simulink model "CustArch_v22"  (R2020a)
settings: Solver=FixedStepDiscrete  StartTime=0.0  StopTime=840000  RelTol=1e-3
undefined symbols (not defined in the file): closed_loop_neuroscience, sqrt_uint32
libraries: hdlsllib x107, simulink x104
(part 2 of 3)

== system CustArch_v22/cust_architecture/process_and_retrieve/spike_detection/LocalMaximaAdaptiveThreshold ==
  filter_output : Inport
  InputState : Inport  Port=2
  write porcessing addr = read from storage addr +1 : Inport  Port=3
  LocalMaxima : Subsystem
  RMS_computation : Subsystem
  local_maxima_out : Outport
  wires:
  filter_output/1 -> RMS_computation/1(filter_output), LocalMaxima/2(filter_output)
  InputState/1 -> RMS_computation/3(InputState), LocalMaxima/3(InputState)
  write porcessing addr = read from storage addr +1/1 -> RMS_computation/2(write porcessing addr = read from storage addr +1), LocalMaxima/4(write porcessing addr = read from storage addr +1)
  LocalMaxima/1(Out1) -> local_maxima_out/1
  RMS_computation/1(adaptive_th) -> LocalMaxima/1(adaptive_th)

== system CustArch_v22/cust_architecture/process_and_retrieve/spike_detection/refractory_period ==
  InputState : Inport
  wr_en : Inport  Port=2
  write porcessing addr = read from storage addr +1 : Inport  Port=3
  rd_addr : Inport  Port=4
  Constant : Constant  OutDataTypeStr=uint16  SampleTime=-1
  Constant1 : Constant  Value=0  OutDataTypeStr=uint16  SampleTime=-1
  Delay : Delay  DelayLength=1  InitialCondition=0
  HDL Counter : hdlsllib/Sources/HDL Counter  CountType=Free running  CountInit=0  CountStep=1  CountMax=2^32  CountFromType=Initial value  CountFrom=0  CountResetPort=off  CountLoadPort=off  CountEnbPort=on  CountDirPort=off  CountDataType=Unsigned  CountWordLen=32  CountFracLen=0  CountSampTime=1
  Logical Operator : Logic  IconShape=distinctive  AllPortsSameDT=off  OutDataTypeStr=boolean
  Sum : Sum  Inputs=+-
  Switch : Switch  Criteria=u2 > Threshold
  Terminator2 : Terminator
  Terminator3 : Terminator
  input_state_AC : simulink/Logic and Bit Operations/Compare To Constant  relop===  const=1  OutDataTypeStr=boolean
  refractory_period : simulink/Logic and Bit Operations/Compare To Constant  relop=>=  const=30  OutDataTypeStr=boolean
  spikes : hdlsllib/HDL RAMs/Dual Port RAM  ram_size=9
      settings: SourceProductBaseCode=SL
  timestamp_before : hdlsllib/HDL RAMs/Dual Port RAM  ram_size=9
      settings: SourceProductBaseCode=SL
  refractory_check : Outport
  spike : Outport  Port=2
  wires:
  timestamp_before/1 -> Terminator2/1
  Delay/1 -> spikes/2, timestamp_before/2
  spikes/2 -> spike/1
  write porcessing addr = read from storage addr +1/1 -> input_state_AC/1, Delay/1, timestamp_before/4
  wr_en/1 -> Switch/2, timestamp_before/3
  timestamp_before/2 -> Sum/2
  rd_addr/1 -> spikes/4
  spikes/1 -> Terminator3/1
  Sum/1 -> refractory_period/1
  InputState/1 -> spikes/3, Logical Operator/2  "read from porcessing"
  refractory_period/1 -> Logical Operator/1
  Logical Operator/1 -> refractory_check/1
  input_state_AC/1 -> HDL Counter/1  "read from porcessing"
  HDL Counter/1 -> timestamp_before/1, Sum/1
  Constant/1 -> Switch/1
  Switch/1 -> spikes/1
  Constant1/1 -> Switch/3

== system CustArch_v22/cust_architecture/input_interpret_store_retrieve/Interpret_to_RAM_input/interpret incoming data/condition to count DAC or ADC  ==
  fifo_write_to : Inport
  input_state : Inport  Port=2
  AND : Logic  IconShape=distinctive  AllPortsSameDT=off  OutDataTypeStr=boolean
  OR : Logic  Operator=OR  IconShape=distinctive  AllPortsSameDT=off  OutDataTypeStr=boolean
  is state_ADC : simulink/Logic and Bit Operations/Compare To Constant  relop===  const=13  OutDataTypeStr=boolean
  is state_DAC : simulink/Logic and Bit Operations/Compare To Constant  relop===  const=12  OutDataTypeStr=boolean
  Out1 : Outport  VectorParamsAs1DForOutWhenUnconnected=off
  wires:
  input_state/1 -> is state_DAC/1, is state_ADC/1
  is state_DAC/1 -> OR/1
  is state_ADC/1 -> OR/2
  fifo_write_to/1 -> AND/1
  OR/1 -> AND/2
  AND/1 -> Out1/1

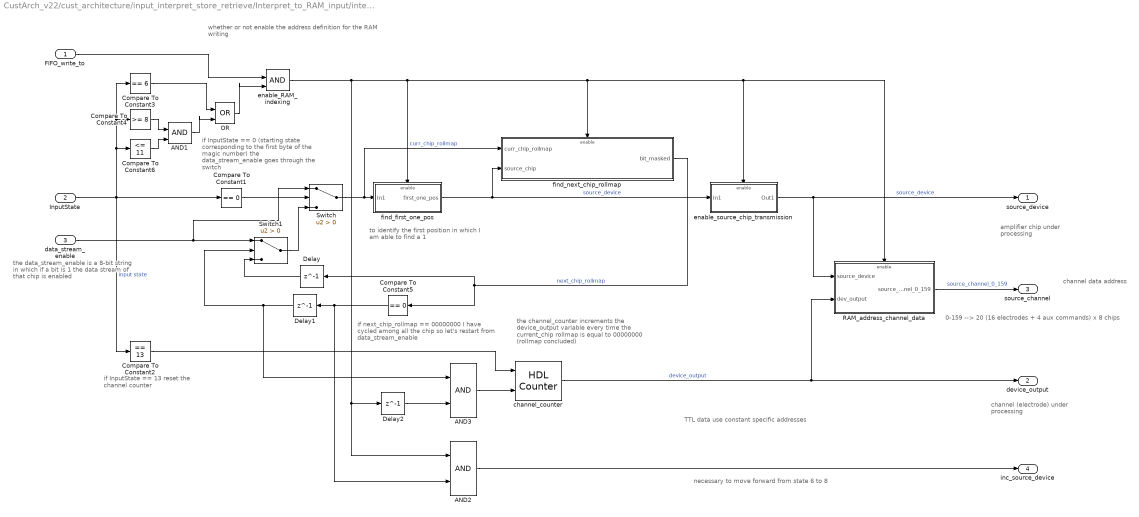
== system CustArch_v22/cust_architecture/input_interpret_store_retrieve/Interpret_to_RAM_input/interpret incoming data/get_sources_and_RAM_addresses ==
  note: necessary to move forward from state 6 to 8
  note: amplifier chip under
      | processing
  note: the channel_counter increments the
      | device_output variable every time the
      | current_chip rollmap is equal to 00000000
      | (rollmap concluded)
  note: if InputState == 13
      | reset the channel counter
  note: whether or not enable the address definition
      | for the RAM writing
  note: if InputState == 0 (starting state corresponding to the first byte
      | of the magic number) the data_stream_enable goes through the switch
  note: 0-159 --> 20 (16 electrodes + 4 aux commands) x 8 chips
  note: to identify the first position in which
      | I am able to find a 1
  note: if next_chip_rollmap == 00000000 I have cycled among all the chip so let's restart from data_stream_enable
  note: the data_stream_enable is a 8-bit string in which if a bit is 1 the data stream of that chip is enabled
  note: channel (electrode) under
      | processing
  note: channel data
      | address
  note: TTL data use constant specific addresses
  FIFO_write_to : Inport
  InputState : Inport  Port=2
  data_stream_enable : Inport  Port=3
  AND1 : Logic  IconShape=distinctive  AllPortsSameDT=off  OutDataTypeStr=boolean
  AND2 : Logic  IconShape=distinctive  AllPortsSameDT=off  OutDataTypeStr=boolean
  AND3 : Logic  IconShape=distinctive  AllPortsSameDT=off  OutDataTypeStr=boolean
  Compare To Constant1 : simulink/Logic and Bit Operations/Compare To Constant  relop===  const=0  OutDataTypeStr=boolean
  Compare To Constant2 : simulink/Logic and Bit Operations/Compare To Constant  relop===  const=13  OutDataTypeStr=boolean
  Compare To Constant3 : simulink/Logic and Bit Operations/Compare To Constant  relop===  const=6  OutDataTypeStr=boolean
  Compare To Constant4 : simulink/Logic and Bit Operations/Compare To Constant  relop=>=  const=8  OutDataTypeStr=boolean
  Compare To Constant5 : simulink/Logic and Bit Operations/Compare To Constant  relop===  const=0  OutDataTypeStr=boolean
  Compare To Constant6 : simulink/Logic and Bit Operations/Compare To Constant  relop=<=  const=11  OutDataTypeStr=boolean
  Delay : Delay  DelayLength=1  InitialCondition=0
  Delay1 : Delay  DelayLength=1  InitialCondition=0
  Delay2 : Delay  DelayLength=1  InitialCondition=0
  OR : Logic  Operator=OR  IconShape=distinctive  AllPortsSameDT=off  OutDataTypeStr=boolean
  RAM_address_channel_data : Subsystem
  Switch : Switch  Criteria=u2 > Threshold  OutDataTypeStr=uint8
  Switch1 : Switch  Criteria=u2 > Threshold
  channel_counter : hdlsllib/Sources/HDL Counter  CountType=Count limited  CountInit=0  CountStep=1  CountMax=20  CountFromType=Specify  CountFrom=0  CountResetPort=on  CountLoadPort=off  CountEnbPort=on  CountDirPort=off  CountDataType=Unsigned  CountWordLen=8  CountFracLen=0  CountSampTime=1
  enable_RAM_indexing : Logic  IconShape=distinctive  AllPortsSameDT=off  OutDataTypeStr=boolean
  enable_source_chip_transmission : Subsystem  TreatAsAtomicUnit=on
  find_first_one_pos : Subsystem
  find_next_chip_rollmap : Subsystem
  source_device : Outport  VectorParamsAs1DForOutWhenUnconnected=off
  device_output : Outport  Port=2  VectorParamsAs1DForOutWhenUnconnected=off
  source_channel : Outport  Port=3  VectorParamsAs1DForOutWhenUnconnected=off
  inc_source_device : Outport  Port=4  VectorParamsAs1DForOutWhenUnconnected=off
  wires:
  InputState/1 -> Compare To Constant1/1, Compare To Constant2/1, Compare To Constant6/1, Compare To Constant4/1, Compare To Constant3/1  "input state"
  Switch/1 -> find_next_chip_rollmap/1(curr_chip_rollmap), find_first_one_pos/1(In1)  "curr_chip_rollmap"
  Compare To Constant1/1 -> Switch/2
  data_stream_enable/1 -> Switch1/1, Switch/1
  find_next_chip_rollmap/1(bit_masked) -> Delay/1, Compare To Constant5/1  "next_chip_rollmap"
  FIFO_write_to/1 -> enable_RAM_indexing/1
  enable_RAM_indexing/1 -> enable_source_chip_transmission/Enable, RAM_address_channel_data/Enable, find_next_chip_rollmap/Enable, find_first_one_pos/Enable, Delay2/1, AND2/1
  Switch1/1 -> Switch/3
  Compare To Constant5/1 -> Delay1/1, AND2/2
  channel_counter/1 -> device_output/1, RAM_address_channel_data/2(dev_output)  "device_output"
  AND3/1 -> channel_counter/2
  Delay/1 -> Switch1/3
  Delay2/1 -> AND3/2
  enable_source_chip_transmission/1(Out1) -> source_device/1, RAM_address_channel_data/1(source_device)  "source_device"
  Compare To Constant3/1 -> OR/1
  RAM_address_channel_data/1(source_channel_0_159) -> source_channel/1  "source_channel_0_159"
  Compare To Constant2/1 -> channel_counter/1
  Compare To Constant4/1 -> AND1/1
  Compare To Constant6/1 -> AND1/2
  AND1/1 -> OR/2
  OR/1 -> enable_RAM_indexing/2
  Delay1/1 -> AND3/1, Switch1/2
  AND2/1 -> inc_source_device/1
  find_first_one_pos/1(first_one_pos) -> enable_source_chip_transmission/1(In1), find_next_chip_rollmap/2(source_chip)  "source_device"

== system CustArch_v22/cust_architecture/output_interpret/Interpret_to_RAM_output/get_enabled_timings /find_next_chip_rollmap ==
  note: this is to identify the next chip for decoding process
  note: bit rotation --> circular rotation of the data_stream_enable 8-bit string
      |
      | Example: data_stream_enable == 01001000
      | right rotation length 1 --> 00100100
      | right rotation length 3 --> 10000100
  In1 : Inport
  Trigger : TriggerPort  VariantControl=Variant
  Bit Rotate : hdlsllib/Logic and Bit Operations/Bit Rotate  mode=Rotate Right  N=1
      settings: SourceProductBaseCode=SL
  Out1 : Outport  InitialOutput=0  VectorParamsAs1DForOutWhenUnconnected=off
  wires:
  In1/1 -> Bit Rotate/1
  Bit Rotate/1 -> Out1/1

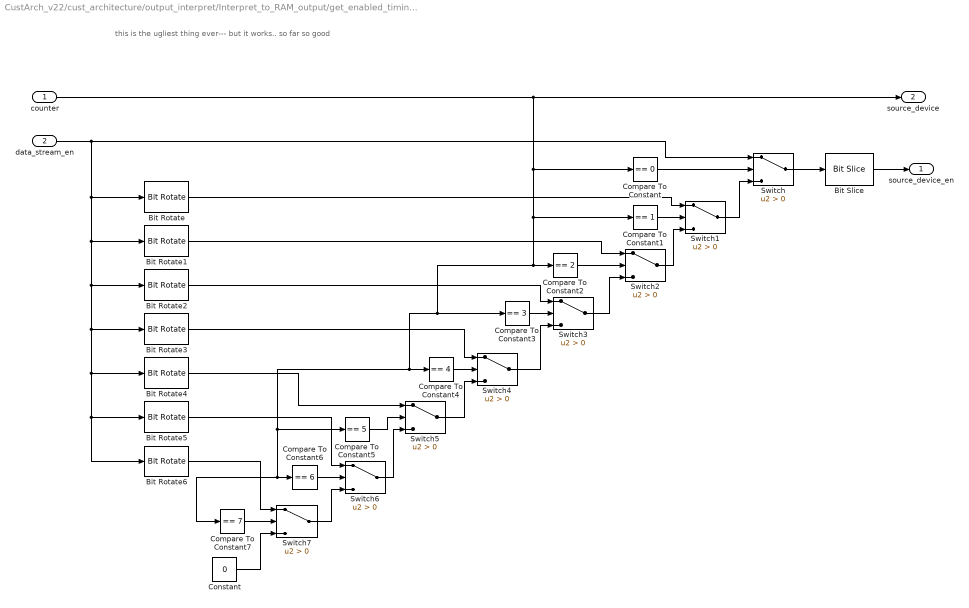
== system CustArch_v22/cust_architecture/output_interpret/Interpret_to_RAM_output/get_enabled_timings /reading_address ==
  note: this is the ugliest thing ever--- but it works.. so far so good
  "counter " : Inport
  data_stream_en : Inport  Port=2
  Bit Rotate : hdlsllib/Logic and Bit Operations/Bit Rotate  mode=Rotate Right  N=1
      settings: SourceProductBaseCode=SL
  Bit Rotate1 : hdlsllib/Logic and Bit Operations/Bit Rotate  mode=Rotate Right  N=2
      settings: SourceProductBaseCode=SL
  Bit Rotate2 : hdlsllib/Logic and Bit Operations/Bit Rotate  mode=Rotate Right  N=3
      settings: SourceProductBaseCode=SL
  Bit Rotate3 : hdlsllib/Logic and Bit Operations/Bit Rotate  mode=Rotate Right  N=4
      settings: SourceProductBaseCode=SL
  Bit Rotate4 : hdlsllib/Logic and Bit Operations/Bit Rotate  mode=Rotate Right  N=5
      settings: SourceProductBaseCode=SL
  Bit Rotate5 : hdlsllib/Logic and Bit Operations/Bit Rotate  mode=Rotate Right  N=6
      settings: SourceProductBaseCode=SL
  Bit Rotate6 : hdlsllib/Logic and Bit Operations/Bit Rotate  mode=Rotate Right  N=7
      settings: SourceProductBaseCode=SL
  Bit Slice : hdlsllib/Logic and Bit Operations/Bit Slice  lidx=0  ridx=0
      settings: SourceProductBaseCode=SL
  Compare To Constant : simulink/Logic and Bit Operations/Compare To Constant  relop===  const=0  OutDataTypeStr=boolean
  Compare To Constant1 : simulink/Logic and Bit Operations/Compare To Constant  relop===  const=1  OutDataTypeStr=boolean
  Compare To Constant2 : simulink/Logic and Bit Operations/Compare To Constant  relop===  const=2  OutDataTypeStr=boolean
  Compare To Constant3 : simulink/Logic and Bit Operations/Compare To Constant  relop===  const=3  OutDataTypeStr=boolean
  Compare To Constant4 : simulink/Logic and Bit Operations/Compare To Constant  relop===  const=4  OutDataTypeStr=boolean
  Compare To Constant5 : simulink/Logic and Bit Operations/Compare To Constant  relop===  const=5  OutDataTypeStr=boolean
  Compare To Constant6 : simulink/Logic and Bit Operations/Compare To Constant  relop===  const=6  OutDataTypeStr=boolean
  Compare To Constant7 : simulink/Logic and Bit Operations/Compare To Constant  relop===  const=7  OutDataTypeStr=boolean
  Constant : Constant  Value=0  OutDataTypeStr=uint8  SampleTime=-1
  Switch{,1..7} (8 alike) : Switch  Criteria=u2 > Threshold
  source_device_en : Outport  VectorParamsAs1DForOutWhenUnconnected=off
  source_device : Outport  Port=2  VectorParamsAs1DForOutWhenUnconnected=off
  wires:
  Compare To Constant/1 -> Switch/2
  Compare To Constant1/1 -> Switch1/2
  Bit Rotate/1 -> Switch1/1
  "counter "/1 -> Compare To Constant7/1, Compare To Constant6/1, Compare To Constant5/1, Compare To Constant4/1, Compare To Constant3/1, Compare To Constant2/1, Compare To Constant1/1, Compare To Constant/1, source_device/1
  Switch1/1 -> Switch/3
  Compare To Constant2/1 -> Switch2/2
  Bit Rotate1/1 -> Switch2/1
  Compare To Constant3/1 -> Switch3/2
  Switch3/1 -> Switch2/3
  Bit Rotate2/1 -> Switch3/1
  Compare To Constant4/1 -> Switch4/2
  Switch4/1 -> Switch3/3
  Bit Rotate3/1 -> Switch4/1
  Compare To Constant5/1 -> Switch5/2
  Bit Rotate4/1 -> Switch5/1
  Switch5/1 -> Switch4/3
  Compare To Constant6/1 -> Switch6/2
  Switch6/1 -> Switch5/3
  Bit Rotate5/1 -> Switch6/1
  Compare To Constant7/1 -> Switch7/2
  Switch7/1 -> Switch6/3
  Bit Rotate6/1 -> Switch7/1
  Constant/1 -> Switch7/3
  Switch2/1 -> Switch1/3
  data_stream_en/1 -> Switch/1, Bit Rotate/1, Bit Rotate1/1, Bit Rotate2/1, Bit Rotate3/1, Bit Rotate4/1, Bit Rotate5/1, Bit Rotate6/1
  Switch/1 -> Bit Slice/1
  Bit Slice/1 -> source_device_en/1

== system CustArch_v22/cust_architecture/process_and_retrieve/filtering/two_pole_IIR/HP_Butter_2nd ==
  Input : Inport  OutDataTypeStr=fixdt(1,32,15)
  previous_samples : Inport  Port=2
  Delay{,2,5..7} (5 alike) : Delay  DelayLength=1  InitialCondition=0
  Delay1 : Delay  InitialCondition=0
  Delay3 : Delay  DelayLength=3  InitialCondition=0
  Delay4 : Delay  DelayLength=4  InitialCondition=0
  Demux : Demux  Outputs=2
  SumA21 : Sum  Inputs=|+-  AccumDataTypeStr=fixdt(1,32,6)  OutDataTypeStr=fixdt(1,32,6)  RndMeth=Nearest  SaturateOnIntegerOverflow=on
  SumA31 : Sum  Inputs=|+-  AccumDataTypeStr=fixdt(1,32,6)  OutDataTypeStr=fixdt(1,32,7)  RndMeth=Nearest  SaturateOnIntegerOverflow=on
  SumB21 : Sum  Inputs=|++  AccumDataTypeStr=fixdt(1,32,6)  OutDataTypeStr=fixdt(1,32,7)  RndMeth=Nearest  SaturateOnIntegerOverflow=on
  SumB31 : Sum  Inputs=|++  AccumDataTypeStr=fixdt(1,32,7)  OutDataTypeStr=fixdt(1,32,15)  RndMeth=Nearest  SaturateOnIntegerOverflow=on
  a(2)(1) : Gain  Gain=-1.9111970674260732  ParamDataTypeStr=fixdt(1,32,30)  OutDataTypeStr=fixdt(1,32,6)  RndMeth=Nearest  SaturateOnIntegerOverflow=on
  a(3)(1) : Gain  Gain=0.914975834801433852  ParamDataTypeStr=fixdt(0,32,32)  OutDataTypeStr=fixdt(1,32,8)  RndMeth=Nearest  SaturateOnIntegerOverflow=on
  b(2)(1) : Gain  Gain=-2  ParamDataTypeStr=fixdt(1,32,30)  OutDataTypeStr=fixdt(1,32,6)  RndMeth=Nearest  SaturateOnIntegerOverflow=on
  s(1) : Gain  Gain=0.956543225556876764  ParamDataTypeStr=fixdt(0,32,32)  OutDataTypeStr=fixdt(1,32,16)  RndMeth=Nearest  SaturateOnIntegerOverflow=on
  Output : Outport  OutDataTypeStr=fixdt(1,32,15)
  Output1 : Outport  Port=2
  wires:
  previous_samples/1 -> Demux/1
  SumA31/1 -> Output1/1, Delay2/1
  a(3)(1)/1 -> Delay1/1
  SumB21/1 -> Delay5/1
  b(2)(1)/1 -> Delay3/1
  SumA21/1 -> Delay/1
  a(2)(1)/1 -> Delay7/1
  Input/1 -> s(1)/1
  SumB31/1 -> Output/1
  s(1)/1 -> Delay6/1
  Demux/2 -> Delay4/1, a(3)(1)/1
  Demux/1 -> b(2)(1)/1, a(2)(1)/1
  Delay/1 -> SumA31/1
  Delay1/1 -> SumA31/2
  Delay2/1 -> SumB21/1
  Delay3/1 -> SumB21/2
  Delay4/1 -> SumB31/2
  Delay5/1 -> SumB31/1
  Delay6/1 -> SumA21/1
  Delay7/1 -> SumA21/2

== system CustArch_v22/cust_architecture/process_and_retrieve/spike_detection/LocalMaximaAdaptiveThreshold/LocalMaxima ==
  adaptive_th : Inport
  filter_output : Inport  Port=2
  InputState : Inport  Port=3
  write porcessing addr = read from storage addr +1 : Inport  Port=4
  Delay1 : Delay  DelayLength=1  InitialCondition=0
  Delay2 : Delay  DelayLength=1  InitialCondition=0
  Logical Operator1 : Logic  Inputs=3  IconShape=distinctive  AllPortsSameDT=off  OutDataTypeStr=boolean
  Relational Operator : RelationalOperator  Operator=<  OutDataTypeStr=boolean  RndMeth=Simplest
  Terminator1 : Terminator
  Terminator2 : Terminator
  check_t-1 : RelationalOperator  Operator=<  OutDataTypeStr=boolean  RndMeth=Simplest
  check_t-2 : RelationalOperator  Operator=<  OutDataTypeStr=boolean  RndMeth=Simplest
  sample_t-1 : hdlsllib/HDL RAMs/Dual Port RAM  ram_size=9
      settings: SourceProductBaseCode=SL
  sample_t-2 : hdlsllib/HDL RAMs/Dual Port RAM  ram_size=9
      settings: SourceProductBaseCode=SL
  Out1 : Outport
  wires:
  Delay1/1 -> sample_t-1/2
  Relational Operator/1 -> Logical Operator1/1  "read from porcessing"
  sample_t-1/2 -> sample_t-2/1, Relational Operator/1, check_t-2/1, check_t-1/1
  check_t-2/1 -> Logical Operator1/3
  sample_t-2/2 -> check_t-1/2
  filter_output/1 -> sample_t-1/1, check_t-2/2
  sample_t-1/1 -> Terminator2/1
  write porcessing addr = read from storage addr +1/1 -> sample_t-2/4, Delay2/1, Delay1/1, sample_t-1/4
  sample_t-2/1 -> Terminator1/1
  check_t-1/1 -> Logical Operator1/2
  Delay2/1 -> sample_t-2/2
  InputState/1 -> sample_t-2/3, sample_t-1/3
  Logical Operator1/1 -> Out1/1
  adaptive_th/1 -> Relational Operator/2

== system CustArch_v22/cust_architecture/process_and_retrieve/spike_detection/LocalMaximaAdaptiveThreshold/RMS_computation ==
  filter_output : Inport
  write porcessing addr = read from storage addr +1 : Inport  Port=2
  InputState : Inport  Port=3
  Delay1 : Delay  DelayLength=1  InitialCondition=0
  Delay2 : Delay  DelayLength=20  InitialCondition=0
  Delay3 : Delay  DelayLength=1  InitialCondition=0
  Delay4 : Delay  DelayLength=21  InitialCondition=0
  Product : Product
  Sum : Sum  Inputs=++|  OutDataTypeStr=uint64
  Switch : Switch  Criteria=u2 > Threshold  OutDataTypeStr=uint64
  Terminator3 : Terminator
  Terminator4 : Terminator
  adaptive_th_computation : Subsystem
  buffer_counter : Subsystem
  count rst : Constant  Value=0  OutDataTypeStr=uint64  SampleTime=-1
  n : Gain  Gain=1/2  OutDataTypeStr=uint32
  sqrt : Subsystem
  square_sum : hdlsllib/HDL RAMs/Dual Port RAM  ram_size=9
      settings: SourceProductBaseCode=SL
  th : hdlsllib/HDL RAMs/Dual Port RAM  ram_size=9
      settings: SourceProductBaseCode=SL
  adaptive_th : Outport
  wires:
  count rst/1 -> Switch/1
  square_sum/2 -> n/1, Switch/3  "square_sum"
  Sum/1 -> square_sum/1
  th/1 -> Terminator3/1
  Product/1 -> Sum/2
  Delay4/1 -> th/2
  Switch/1 -> Sum/1
  Delay3/1 -> square_sum/2
  square_sum/1 -> Terminator4/1
  InputState/1 -> square_sum/3, buffer_counter/1(InputState)
  filter_output/1 -> Product/2, Product/1  "filter_out"
  th/2 -> adaptive_th/1
  adaptive_th_computation/1(Out1) -> th/1  "adaptive_th"
  buffer_counter/1(Out1) -> Delay2/1, Switch/2
  n/1 -> Delay1/1  "rms"
  sqrt/1(rms) -> adaptive_th_computation/1(u)  "rms"
  Delay1/1 -> sqrt/1(square_sum_n)
  Delay2/1 -> th/3
  write porcessing addr = read from storage addr +1/1 -> buffer_counter/2(write porcessing addr = read from storage addr +1), Delay3/1, square_sum/4, th/4, Delay4/1

== system CustArch_v22/cust_architecture/input_interpret_store_retrieve/Interpret_to_RAM_input/interpret incoming data/get_sources_and_RAM_addresses/RAM_address_channel_data ==
  note: channel data address codification
      | according to this table
  source_device : Inport
  dev_output : Inport  Port=2
  Enable : EnablePort
  Bit Concat : hdlsllib/Logic and Bit Operations/Bit Concat  numInputs=2  mask(Bit Concat){}
      mask Display: image('C:\Users\diflo\OneDrive - Fondazione Istituto Italiano Tecnologia\Progetto MathWorks\Project\Documentation\Images\Simulink\source_channel_0_159.png'); % Use "Edit Image" on toolstrip to change.
  Bit Slice : hdlsllib/Logic and Bit Operations/Bit Slice  lidx=4  ridx=0
      settings: SourceProductBaseCode=SL
  Bit Slice1 : hdlsllib/Logic and Bit Operations/Bit Slice  lidx=2  ridx=0
      settings: SourceProductBaseCode=SL
  source_channel_0_159 : Outport  InitialOutput=0  VectorParamsAs1DForOutWhenUnconnected=off
  wires:
  source_device/1 -> Bit Slice1/1
  Bit Slice/1 -> Bit Concat/1
  Bit Slice1/1 -> Bit Concat/2
  Bit Concat/1 -> source_channel_0_159/1  "source_channel_0_159"
  dev_output/1 -> Bit Slice/1

== system CustArch_v22/cust_architecture/input_interpret_store_retrieve/Interpret_to_RAM_input/interpret incoming data/get_sources_and_RAM_addresses/enable_source_chip_transmission ==
  In1 : Inport
  Enable : EnablePort
  Out1 : Outport  InitialOutput=0  VectorParamsAs1DForOutWhenUnconnected=off
  wires:
  In1/1 -> Out1/1

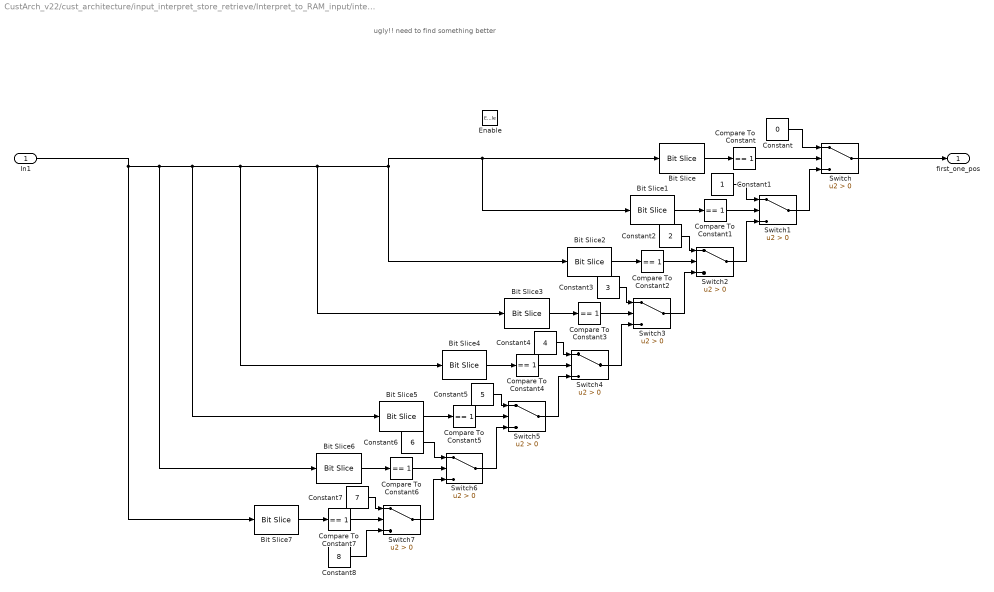
== system CustArch_v22/cust_architecture/input_interpret_store_retrieve/Interpret_to_RAM_input/interpret incoming data/get_sources_and_RAM_addresses/find_first_one_pos ==
  note: ugly!! need to find something better
  In1 : Inport
  Enable : EnablePort
  Bit Slice : hdlsllib/Logic and Bit Operations/Bit Slice  lidx=0  ridx=0
      settings: SourceProductBaseCode=SL
  Bit Slice1 : hdlsllib/Logic and Bit Operations/Bit Slice  lidx=1  ridx=1
      settings: SourceProductBaseCode=SL
  Bit Slice2 : hdlsllib/Logic and Bit Operations/Bit Slice  lidx=2  ridx=2
      settings: SourceProductBaseCode=SL
  Bit Slice3 : hdlsllib/Logic and Bit Operations/Bit Slice  lidx=3  ridx=3
      settings: SourceProductBaseCode=SL
  Bit Slice4 : hdlsllib/Logic and Bit Operations/Bit Slice  lidx=4  ridx=4
      settings: SourceProductBaseCode=SL
  Bit Slice5 : hdlsllib/Logic and Bit Operations/Bit Slice  lidx=5  ridx=5
      settings: SourceProductBaseCode=SL
  Bit Slice6 : hdlsllib/Logic and Bit Operations/Bit Slice  lidx=6  ridx=6
      settings: SourceProductBaseCode=SL
  Bit Slice7 : hdlsllib/Logic and Bit Operations/Bit Slice  lidx=7  ridx=7
      settings: SourceProductBaseCode=SL
  Compare To Constant{,1..7} (8 alike) : simulink/Logic and Bit Operations/Compare To Constant  relop===  const=1  OutDataTypeStr=boolean
  Constant : Constant  Value=0  OutDataTypeStr=uint8  SampleTime=-1
  Constant1 : Constant  OutDataTypeStr=uint8  SampleTime=-1
  Constant2 : Constant  Value=2  OutDataTypeStr=uint8  SampleTime=-1
  Constant3 : Constant  Value=3  OutDataTypeStr=uint8  SampleTime=-1
  Constant4 : Constant  Value=4  OutDataTypeStr=uint8  SampleTime=-1
  Constant5 : Constant  Value=5  OutDataTypeStr=uint8  SampleTime=-1
  Constant6 : Constant  Value=6  OutDataTypeStr=uint8  SampleTime=-1
  Constant7 : Constant  Value=7  OutDataTypeStr=uint8  SampleTime=-1
  Constant8 : Constant  Value=8  OutDataTypeStr=uint8  SampleTime=-1
  Switch{,1..7} (8 alike) : Switch  Criteria=u2 > Threshold
  first_one_pos : Outport  InitialOutput=0  VectorParamsAs1DForOutWhenUnconnected=off
  wires:
  Compare To Constant/1 -> Switch/2
  Bit Slice/1 -> Compare To Constant/1
  Switch/1 -> first_one_pos/1
  Bit Slice1/1 -> Compare To Constant1/1
  Switch1/1 -> Switch/3
  Compare To Constant1/1 -> Switch1/2
  Bit Slice2/1 -> Compare To Constant2/1
  Compare To Constant2/1 -> Switch2/2
  Switch2/1 -> Switch1/3
  Bit Slice3/1 -> Compare To Constant3/1
  Compare To Constant3/1 -> Switch3/2
  Switch3/1 -> Switch2/3
  Switch4/1 -> Switch3/3
  Bit Slice4/1 -> Compare To Constant4/1
  Compare To Constant4/1 -> Switch4/2
  Bit Slice5/1 -> Compare To Constant5/1
  Compare To Constant5/1 -> Switch5/2
  Switch5/1 -> Switch4/3
  Bit Slice6/1 -> Compare To Constant6/1
  Compare To Constant6/1 -> Switch6/2
  Switch6/1 -> Switch5/3
  Switch7/1 -> Switch6/3
  Compare To Constant7/1 -> Switch7/2
  Bit Slice7/1 -> Compare To Constant7/1
  Constant/1 -> Switch/1
  Constant1/1 -> Switch1/1
  Constant2/1 -> Switch2/1
  Constant3/1 -> Switch3/1
  Constant4/1 -> Switch4/1
  Constant5/1 -> Switch5/1
  Constant6/1 -> Switch6/1
  Constant7/1 -> Switch7/1
  Constant8/1 -> Switch7/3
  In1/1 -> Bit Slice7/1, Bit Slice6/1, Bit Slice5/1, Bit Slice4/1, Bit Slice3/1, Bit Slice2/1, Bit Slice1/1, Bit Slice/1

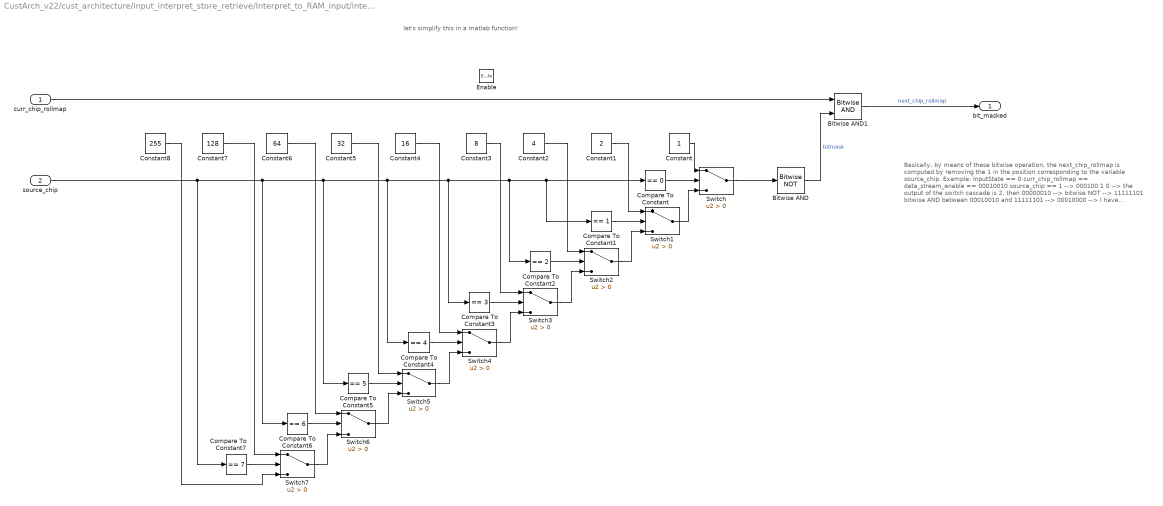
== system CustArch_v22/cust_architecture/input_interpret_store_retrieve/Interpret_to_RAM_input/interpret incoming data/get_sources_and_RAM_addresses/find_next_chip_rollmap ==
  note: Basically, by means of these bitwise operation, the next_chip_rollmap is computed by removing the 1 in the position corresponding to the
      | variable source_chip. Example:
      |
      | InputState == 0
      | curr_chip_rollmap == data_stream_enable == 00010010
      | source_chip == 1 --> 000100 1 0
      |
      | --> the output of the switch cascade is 2, then 00000010 --> bitwise NOT --> 11111101
      |
      | bitwise AND between 00010010 and 11111101 --> 00010000 --> I have removed the 1 corresponding to the position 2! --> ready for the next chip rollmap!
  note: let's simplify this in a matlab function!
  curr_chip_rollmap : Inport
  source_chip : Inport  Port=2
  Enable : EnablePort
  Bitwise AND : simulink/Logic and Bit Operations/Bitwise Operator  logicop=NOT  UseBitMask=off  BitMask=bin2dec('11011001')  BitMaskRealWorld=Stored Integer
  Bitwise AND1 : simulink/Logic and Bit Operations/Bitwise Operator  logicop=AND  UseBitMask=off  NumInputPorts=2  BitMask=bin2dec('11011001')  BitMaskRealWorld=Stored Integer
  Compare To Constant : simulink/Logic and Bit Operations/Compare To Constant  relop===  const=0  OutDataTypeStr=boolean
  Compare To Constant1 : simulink/Logic and Bit Operations/Compare To Constant  relop===  const=1  OutDataTypeStr=boolean
  Compare To Constant2 : simulink/Logic and Bit Operations/Compare To Constant  relop===  const=2  OutDataTypeStr=boolean
  Compare To Constant3 : simulink/Logic and Bit Operations/Compare To Constant  relop===  const=3  OutDataTypeStr=boolean
  Compare To Constant4 : simulink/Logic and Bit Operations/Compare To Constant  relop===  const=4  OutDataTypeStr=boolean
  Compare To Constant5 : simulink/Logic and Bit Operations/Compare To Constant  relop===  const=5  OutDataTypeStr=boolean
  Compare To Constant6 : simulink/Logic and Bit Operations/Compare To Constant  relop===  const=6  OutDataTypeStr=boolean
  Compare To Constant7 : simulink/Logic and Bit Operations/Compare To Constant  relop===  const=7  OutDataTypeStr=boolean
  Constant : Constant  OutDataTypeStr=uint8  SampleTime=-1
  Constant1 : Constant  Value=2  OutDataTypeStr=uint8  SampleTime=-1
  Constant2 : Constant  Value=4  OutDataTypeStr=uint8  SampleTime=-1
  Constant3 : Constant  Value=8  OutDataTypeStr=uint8  SampleTime=-1
  Constant4 : Constant  Value=16  OutDataTypeStr=uint8  SampleTime=-1
  Constant5 : Constant  Value=32  OutDataTypeStr=uint8  SampleTime=-1
  Constant6 : Constant  Value=64  OutDataTypeStr=uint8  SampleTime=-1
  Constant7 : Constant  Value=128  OutDataTypeStr=uint8  SampleTime=-1
  Constant8 : Constant  Value=255  OutDataTypeStr=uint8  SampleTime=-1
  Switch{,1..7} (8 alike) : Switch  Criteria=u2 > Threshold
  bit_masked : Outport  InitialOutput=0  VectorParamsAs1DForOutWhenUnconnected=off
  wires:
  Compare To Constant/1 -> Switch/2
  Constant/1 -> Switch/1
  Switch/1 -> Bitwise AND/1
  Compare To Constant1/1 -> Switch1/2
  Switch1/1 -> Switch/3
  Constant1/1 -> Switch1/1
  Compare To Constant2/1 -> Switch2/2
  Switch2/1 -> Switch1/3
  Constant2/1 -> Switch2/1
  Switch3/1 -> Switch2/3
  Compare To Constant3/1 -> Switch3/2
  Constant3/1 -> Switch3/1
  Compare To Constant4/1 -> Switch4/2
  Switch4/1 -> Switch3/3
  Constant4/1 -> Switch4/1
  Compare To Constant5/1 -> Switch5/2
  Switch5/1 -> Switch4/3
  Constant5/1 -> Switch5/1
  Switch6/1 -> Switch5/3
  Compare To Constant6/1 -> Switch6/2
  Constant6/1 -> Switch6/1
  Switch7/1 -> Switch6/3
  Compare To Constant7/1 -> Switch7/2
  source_chip/1 -> Compare To Constant7/1, Compare To Constant6/1, Compare To Constant5/1, Compare To Constant4/1, Compare To Constant3/1, Compare To Constant2/1, Compare To Constant1/1, Compare To Constant/1
  Constant7/1 -> Switch7/1
  Constant8/1 -> Switch7/3
  Bitwise AND/1 -> Bitwise AND1/2  "bitmask"
  curr_chip_rollmap/1 -> Bitwise AND1/1
  Bitwise AND1/1 -> bit_masked/1  "next_chip_rollmap"

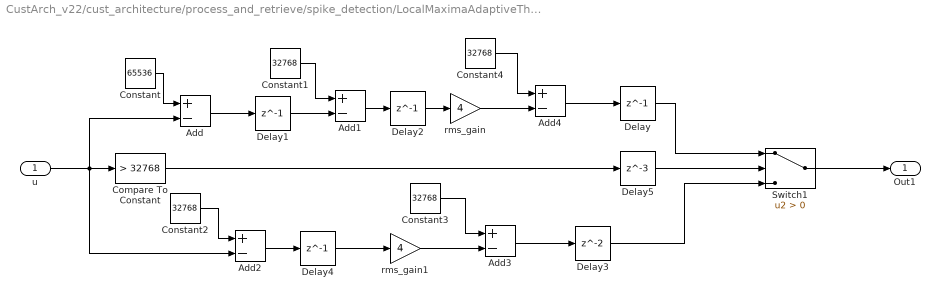
== system CustArch_v22/cust_architecture/process_and_retrieve/spike_detection/LocalMaximaAdaptiveThreshold/RMS_computation/adaptive_th_computation ==
  u : Inport
  Add{,1..4} (5 alike) : Sum  Inputs=+-  OutDataTypeStr=uint16
  Compare To Constant : simulink/Logic and Bit Operations/Compare To Constant  relop=>  const=32768  OutDataTypeStr=boolean
  Constant : Constant  Value=65536  OutDataTypeStr=uint16  SampleTime=-1
  Constant{1..4} (4 alike) : Constant  Value=32768  OutDataTypeStr=uint16  SampleTime=-1
  Delay{,1..2,4} (4 alike) : Delay  DelayLength=1  InitialCondition=0
  Delay3 : Delay  InitialCondition=0
  Delay5 : Delay  DelayLength=3  InitialCondition=0
  Switch1 : Switch  Criteria=u2 > Threshold
  rms_gain : Gain  Gain=4  OutDataTypeStr=uint16
  rms_gain1 : Gain  Gain=4  OutDataTypeStr=uint16
  Out1 : Outport
  wires:
  Add3/1 -> Delay3/1
  Constant2/1 -> Add2/1
  Constant/1 -> Add/1
  Compare To Constant/1 -> Delay5/1
  Add/1 -> Delay1/1
  Constant4/1 -> Add4/1
  rms_gain/1 -> Add4/2
  Constant1/1 -> Add1/1
  Add4/1 -> Delay/1
  rms_gain1/1 -> Add3/2
  Constant3/1 -> Add3/1
  Add2/1 -> Delay4/1
  Add1/1 -> Delay2/1
  u/1 -> Add2/2, Add/2, Compare To Constant/1
  Switch1/1 -> Out1/1
  Delay1/1 -> Add1/2
  Delay/1 -> Switch1/1
  Delay2/1 -> rms_gain/1
  Delay3/1 -> Switch1/3
  Delay4/1 -> rms_gain1/1
  Delay5/1 -> Switch1/2

== system CustArch_v22/cust_architecture/process_and_retrieve/spike_detection/LocalMaximaAdaptiveThreshold/RMS_computation/buffer_counter ==
  InputState : Inport
  write porcessing addr = read from storage addr +1 : Inport  Port=2
  Delay : Delay  DelayLength=1  InitialCondition=0
  Switch : Switch  Criteria=u2 > Threshold  OutDataTypeStr=uint32
  Terminator4 : Terminator
  count_rst : Constant  Value=0  OutDataTypeStr=uint16  SampleTime=-1
  incr : Sum  AccumDataTypeStr=uint32
  rst_check : simulink/Logic and Bit Operations/Compare To Constant  relop===  const=2  OutDataTypeStr=boolean
  square_sum : hdlsllib/HDL RAMs/Dual Port RAM  ram_size=9
      settings: SourceProductBaseCode=SL
  Out1 : Outport
  wires:
  square_sum/2 -> rst_check/1, Switch/3
  square_sum/1 -> Terminator4/1
  count_rst/1 -> Switch/1
  Delay/1 -> square_sum/2
  incr/1 -> square_sum/1
  InputState/1 -> incr/1, square_sum/3
  Switch/1 -> incr/2
  write porcessing addr = read from storage addr +1/1 -> square_sum/4, Delay/1
  rst_check/1 -> Out1/1, Switch/2

== system CustArch_v22/cust_architecture/process_and_retrieve/spike_detection/LocalMaximaAdaptiveThreshold/RMS_computation/sqrt ==
  square_sum_n : Inport
  Data Type Conversion : DataTypeConversion  OutDataTypeStr=uint16
  sqrt_uint32 : Subsystem  AncestorBlock=closed_loop_neuroscience/sqrt_uint32
      mask Display:
      | color('white'); port_label('input',1,'input_data')
      | color('white'); port_label('output',1,'sqrt')
  rms : Outport
  wires:
  Data Type Conversion/1 -> rms/1
  sqrt_uint32/1(sqrt) -> Data Type Conversion/1
  square_sum_n/1 -> sqrt_uint32/1(input_data)

== system CustArch_v22/cust_architecture/process_and_retrieve/spike_detection/LocalMaximaAdaptiveThreshold/RMS_computation/sqrt/sqrt_uint32 ==
  input_data : Inport
  1_32bit : Subsystem
  sqrt : Outport
  wires:
  input_data/1 -> 1_32bit/1(shiftI)
  1_32bit/1(QO) -> sqrt/1

== system CustArch_v22/cust_architecture/process_and_retrieve/spike_detection/LocalMaximaAdaptiveThreshold/RMS_computation/sqrt/sqrt_uint32/1_32bit ==
  shiftI : Inport
  1_start_8bit : Subsystem
  2_8bit : Subsystem
  3_8bit : Subsystem
  4_end_8bit : Subsystem
  QO : Outport
  wires:
  3_8bit/1(shiftO) -> 4_end_8bit/1(shiftI)
  1_start_8bit/1(shiftO) -> 2_8bit/1(shiftI)
  1_start_8bit/2(RO) -> 2_8bit/2(RI)
  1_start_8bit/3(QO) -> 2_8bit/3(QI)
  2_8bit/1(shiftO) -> 3_8bit/1(shiftI)
  3_8bit/2(RO) -> 4_end_8bit/2(RI)
  3_8bit/3(QO) -> 4_end_8bit/3(QI)
  2_8bit/2(RO) -> 3_8bit/2(RI)
  2_8bit/3(QO) -> 3_8bit/3(QI)
  4_end_8bit/1(QO) -> QO/1
  shiftI/1 -> 1_start_8bit/1(shiftI)

== system CustArch_v22/cust_architecture/process_and_retrieve/spike_detection/LocalMaximaAdaptiveThreshold/RMS_computation/sqrt/sqrt_uint32/1_32bit/1_start_8bit ==
  shiftI : Inport
  Subsystem1 : Subsystem
  Subsystem2 : Subsystem
  Subsystem3 : Subsystem
  starting_stage : Subsystem
  shiftO : Outport
  RO : Outport  Port=2
  QO : Outport  Port=3
  wires:
  Subsystem3/2(RO) -> RO/1
  shiftI/1 -> starting_stage/1(shiftI)
  Subsystem3/1(shiftO) -> shiftO/1
  Subsystem2/2(RO) -> Subsystem1/2(RI)
  Subsystem2/1(shiftO) -> Subsystem1/1(shiftI)
  starting_stage/3(QO) -> Subsystem2/3(QI)
  Subsystem3/3(QO) -> QO/1
  Subsystem2/3(QO) -> Subsystem1/3(QI)
  Subsystem1/2(RO) -> Subsystem3/2(RI)
  Subsystem1/1(shiftO) -> Subsystem3/1(shiftI)
  Subsystem1/3(QO) -> Subsystem3/3(QI)
  starting_stage/2(RO) -> Subsystem2/2(RI)
  starting_stage/1(shiftO) -> Subsystem2/1(shiftI)

== system CustArch_v22/cust_architecture/process_and_retrieve/spike_detection/LocalMaximaAdaptiveThreshold/RMS_computation/sqrt/sqrt_uint32/1_32bit/2_8bit ==
  shiftI : Inport
  RI : Inport  Port=2
  QI : Inport  Port=3
  Subsystem1 : Subsystem
  Subsystem2 : Subsystem
  Subsystem3 : Subsystem
  Subsystem4 : Subsystem
  shiftO : Outport
  RO : Outport  Port=2
  QO : Outport  Port=3
  wires:
  QI/1 -> Subsystem2/3(QI)
  shiftI/1 -> Subsystem2/1(shiftI)
  Subsystem4/2(RO) -> RO/1
  Subsystem4/3(QO) -> QO/1
  Subsystem2/1(shiftO) -> Subsystem1/1(shiftI)
  Subsystem1/3(QO) -> Subsystem3/3(QI)
  Subsystem1/2(RO) -> Subsystem3/2(RI)
  RI/1 -> Subsystem2/2(RI)
  Subsystem3/1(shiftO) -> Subsystem4/1(shiftI)
  Subsystem4/1(shiftO) -> shiftO/1
  Subsystem1/1(shiftO) -> Subsystem3/1(shiftI)
  Subsystem3/3(QO) -> Subsystem4/3(QI)
  Subsystem2/2(RO) -> Subsystem1/2(RI)
  Subsystem3/2(RO) -> Subsystem4/2(RI)
  Subsystem2/3(QO) -> Subsystem1/3(QI)

== system CustArch_v22/cust_architecture/process_and_retrieve/spike_detection/LocalMaximaAdaptiveThreshold/RMS_computation/sqrt/sqrt_uint32/1_32bit/3_8bit ==
  shiftI : Inport
  RI : Inport  Port=2
  QI : Inport  Port=3
  Subsystem1 : Subsystem
  Subsystem2 : Subsystem
  Subsystem3 : Subsystem
  Subsystem4 : Subsystem
  shiftO : Outport
  RO : Outport  Port=2
  QO : Outport  Port=3
  wires:
  QI/1 -> Subsystem2/3(QI)
  shiftI/1 -> Subsystem2/1(shiftI)
  Subsystem4/2(RO) -> RO/1
  Subsystem4/3(QO) -> QO/1
  Subsystem2/1(shiftO) -> Subsystem1/1(shiftI)
  Subsystem1/3(QO) -> Subsystem3/3(QI)
  Subsystem1/2(RO) -> Subsystem3/2(RI)
  RI/1 -> Subsystem2/2(RI)
  Subsystem3/1(shiftO) -> Subsystem4/1(shiftI)
  Subsystem4/1(shiftO) -> shiftO/1
  Subsystem1/1(shiftO) -> Subsystem3/1(shiftI)
  Subsystem3/3(QO) -> Subsystem4/3(QI)
  Subsystem2/2(RO) -> Subsystem1/2(RI)
  Subsystem3/2(RO) -> Subsystem4/2(RI)
  Subsystem2/3(QO) -> Subsystem1/3(QI)

== system CustArch_v22/cust_architecture/process_and_retrieve/spike_detection/LocalMaximaAdaptiveThreshold/RMS_computation/sqrt/sqrt_uint32/1_32bit/4_end_8bit ==
  shiftI : Inport
  RI : Inport  Port=2
  QI : Inport  Port=3
  Subsystem1 : Subsystem
  Subsystem2 : Subsystem
  Subsystem3 : Subsystem
  terminal_stage : Subsystem
  QO : Outport
  wires:
  QI/1 -> Subsystem2/3(QI)
  shiftI/1 -> Subsystem2/1(shiftI)
  terminal_stage/1(QO) -> QO/1
  Subsystem2/1(shiftO) -> Subsystem1/1(shiftI)
  Subsystem1/3(QO) -> Subsystem3/3(QI)
  Subsystem1/2(RO) -> Subsystem3/2(RI)
  RI/1 -> Subsystem2/2(RI)
  Subsystem3/1(shiftO) -> terminal_stage/1(shiftI)
  Subsystem1/1(shiftO) -> Subsystem3/1(shiftI)
  Subsystem3/3(QO) -> terminal_stage/3(QI)
  Subsystem2/2(RO) -> Subsystem1/2(RI)
  Subsystem3/2(RO) -> terminal_stage/2(RI)
  Subsystem2/3(QO) -> Subsystem1/3(QI)

== system CustArch_v22/cust_architecture/process_and_retrieve/spike_detection/LocalMaximaAdaptiveThreshold/RMS_computation/sqrt/sqrt_uint32/1_32bit/1_start_8bit/Subsystem1 ==
  shiftI : Inport
  RI : Inport  Port=2
  QI : Inport  Port=3
  Bit Concat5 : hdlsllib/Logic and Bit Operations/Bit Concat  numInputs=2
  Bit Concat8 : hdlsllib/Logic and Bit Operations/Bit Concat  numInputs=3
  Bit Concat9 : hdlsllib/Logic and Bit Operations/Bit Concat  numInputs=2
  Constant13 : Constant  Value=0  OutDataTypeStr=fixdt(0,1,0)  SampleTime=-1
  Constant14 : Constant  Value=0  OutDataTypeStr=fixdt(0,1,0)  SampleTime=-1
  Constant15 : Constant  OutDataTypeStr=fixdt(0,2,0)  SampleTime=-1
  Constant16 : Constant  OutDataTypeStr=fixdt(0,1,0)  SampleTime=-1
  Delay : Delay  DelayLength=1  InitialCondition=0
  Delay5 : Delay  DelayLength=1  InitialCondition=0
  Delay6 : Delay  DelayLength=1  InitialCondition=0
  Extract Bits3 : simulink/Logic and Bit Operations/Extract Bits  bitsToExtract=Range starting with most significant bit  numBits=2  bitIdxRange=[6 7]  outScalingMode=Treat bit field as an integer
  Relational Operator4 : RelationalOperator  OutDataTypeStr=boolean  RndMeth=Simplest
  Shift Arithmetic7 : ArithShift  BitShiftNumber=2  BitShiftDirection=Left
  Subtract4 : Sum  Inputs=+-  OutDataTypeStr=Inherit: Inherit via back propagation
  Switch8 : Switch  Criteria=u2 > Threshold
  Switch9 : Switch  Criteria=u2 > Threshold
  shiftO : Outport
  RO : Outport  Port=2
  QO : Outport  Port=3
  wires:
  Delay6/1 -> QO/1
  Delay5/1 -> RO/1
  Delay/1 -> shiftO/1
  Shift Arithmetic7/1 -> Extract Bits3/1, Delay/1
  Bit Concat5/1 -> Relational Operator4/1, Subtract4/1, Switch8/3
  Subtract4/1 -> Switch8/1
  Relational Operator4/1 -> Switch8/2, Switch9/2
  Bit Concat8/1 -> Delay6/1
  Switch8/1 -> Delay5/1
  RI/1 -> Bit Concat5/1
  Constant16/1 -> Switch9/1
  Constant13/1 -> Switch9/3
  Extract Bits3/1 -> Bit Concat5/2
  Bit Concat9/1 -> Relational Operator4/2, Subtract4/2
  Constant14/1 -> Bit Concat8/1
  shiftI/1 -> Shift Arithmetic7/1
  Constant15/1 -> Bit Concat9/2
  QI/1 -> Bit Concat9/1, Bit Concat8/2
  Switch9/1 -> Bit Concat8/3

== system CustArch_v22/cust_architecture/process_and_retrieve/spike_detection/LocalMaximaAdaptiveThreshold/RMS_computation/sqrt/sqrt_uint32/1_32bit/1_start_8bit/Subsystem2 ==
  shiftI : Inport
  RI : Inport  Port=2
  QI : Inport  Port=3
  Bit Concat5 : hdlsllib/Logic and Bit Operations/Bit Concat  numInputs=2
  Bit Concat8 : hdlsllib/Logic and Bit Operations/Bit Concat  numInputs=3
  Bit Concat9 : hdlsllib/Logic and Bit Operations/Bit Concat  numInputs=2
  Constant13 : Constant  Value=0  OutDataTypeStr=fixdt(0,1,0)  SampleTime=-1
  Constant14 : Constant  Value=0  OutDataTypeStr=fixdt(0,1,0)  SampleTime=-1
  Constant15 : Constant  OutDataTypeStr=fixdt(0,2,0)  SampleTime=-1
  Constant16 : Constant  OutDataTypeStr=fixdt(0,1,0)  SampleTime=-1
  Delay : Delay  DelayLength=1  InitialCondition=0
  Delay5 : Delay  DelayLength=1  InitialCondition=0
  Delay6 : Delay  DelayLength=1  InitialCondition=0
  Extract Bits3 : simulink/Logic and Bit Operations/Extract Bits  bitsToExtract=Range starting with most significant bit  numBits=2  bitIdxRange=[6 7]  outScalingMode=Treat bit field as an integer
  Relational Operator4 : RelationalOperator  OutDataTypeStr=boolean  RndMeth=Simplest
  Shift Arithmetic7 : ArithShift  BitShiftNumber=2  BitShiftDirection=Left
  Subtract4 : Sum  Inputs=+-  OutDataTypeStr=Inherit: Inherit via back propagation
  Switch8 : Switch  Criteria=u2 > Threshold
  Switch9 : Switch  Criteria=u2 > Threshold
  shiftO : Outport
  RO : Outport  Port=2
  QO : Outport  Port=3
  wires:
  Delay6/1 -> QO/1
  Delay5/1 -> RO/1
  Delay/1 -> shiftO/1
  Shift Arithmetic7/1 -> Extract Bits3/1, Delay/1
  Bit Concat5/1 -> Relational Operator4/1, Subtract4/1, Switch8/3
  Subtract4/1 -> Switch8/1
  Relational Operator4/1 -> Switch8/2, Switch9/2
  Bit Concat8/1 -> Delay6/1
  Switch8/1 -> Delay5/1
  RI/1 -> Bit Concat5/1
  Constant16/1 -> Switch9/1
  Constant13/1 -> Switch9/3
  Extract Bits3/1 -> Bit Concat5/2
  Bit Concat9/1 -> Relational Operator4/2, Subtract4/2
  Constant14/1 -> Bit Concat8/1
  shiftI/1 -> Shift Arithmetic7/1
  Constant15/1 -> Bit Concat9/2
  QI/1 -> Bit Concat9/1, Bit Concat8/2
  Switch9/1 -> Bit Concat8/3

== system CustArch_v22/cust_architecture/process_and_retrieve/spike_detection/LocalMaximaAdaptiveThreshold/RMS_computation/sqrt/sqrt_uint32/1_32bit/1_start_8bit/Subsystem3 ==
  shiftI : Inport
  RI : Inport  Port=2
  QI : Inport  Port=3
  Bit Concat5 : hdlsllib/Logic and Bit Operations/Bit Concat  numInputs=2
  Bit Concat8 : hdlsllib/Logic and Bit Operations/Bit Concat  numInputs=3
  Bit Concat9 : hdlsllib/Logic and Bit Operations/Bit Concat  numInputs=2
  Constant13 : Constant  Value=0  OutDataTypeStr=fixdt(0,1,0)  SampleTime=-1
  Constant14 : Constant  Value=0  OutDataTypeStr=fixdt(0,1,0)  SampleTime=-1
  Constant15 : Constant  OutDataTypeStr=fixdt(0,2,0)  SampleTime=-1
  Constant16 : Constant  OutDataTypeStr=fixdt(0,1,0)  SampleTime=-1
  Delay : Delay  DelayLength=1  InitialCondition=0
  Delay5 : Delay  DelayLength=1  InitialCondition=0
  Delay6 : Delay  DelayLength=1  InitialCondition=0
  Extract Bits3 : simulink/Logic and Bit Operations/Extract Bits  bitsToExtract=Range starting with most significant bit  numBits=2  bitIdxRange=[6 7]  outScalingMode=Treat bit field as an integer
  Relational Operator4 : RelationalOperator  OutDataTypeStr=boolean  RndMeth=Simplest
  Shift Arithmetic7 : ArithShift  BitShiftNumber=2  BitShiftDirection=Left
  Subtract4 : Sum  Inputs=+-  OutDataTypeStr=Inherit: Inherit via back propagation
  Switch8 : Switch  Criteria=u2 > Threshold
  Switch9 : Switch  Criteria=u2 > Threshold
  shiftO : Outport
  RO : Outport  Port=2
  QO : Outport  Port=3
  wires:
  Delay6/1 -> QO/1
  Delay5/1 -> RO/1
  Delay/1 -> shiftO/1
  Shift Arithmetic7/1 -> Extract Bits3/1, Delay/1
  Bit Concat5/1 -> Relational Operator4/1, Subtract4/1, Switch8/3
  Subtract4/1 -> Switch8/1
  Relational Operator4/1 -> Switch8/2, Switch9/2
  Bit Concat8/1 -> Delay6/1
  Switch8/1 -> Delay5/1
  RI/1 -> Bit Concat5/1
  Constant16/1 -> Switch9/1
  Constant13/1 -> Switch9/3
  Extract Bits3/1 -> Bit Concat5/2
  Bit Concat9/1 -> Relational Operator4/2, Subtract4/2
  Constant14/1 -> Bit Concat8/1
  shiftI/1 -> Shift Arithmetic7/1
  Constant15/1 -> Bit Concat9/2
  QI/1 -> Bit Concat9/1, Bit Concat8/2
  Switch9/1 -> Bit Concat8/3

== system CustArch_v22/cust_architecture/process_and_retrieve/spike_detection/LocalMaximaAdaptiveThreshold/RMS_computation/sqrt/sqrt_uint32/1_32bit/1_start_8bit/starting_stage ==
  shiftI : Inport
  Bit Concat1 : hdlsllib/Logic and Bit Operations/Bit Concat  numInputs=2
  Constant1 : Constant  OutDataTypeStr=fixdt(0,2,0)  SampleTime=-1
  Constant2 : Constant  OutDataTypeStr=fixdt(0,1)  SampleTime=-1
  Constant3 : Constant  Value=0  OutDataTypeStr=fixdt(0,1,0)  SampleTime=-1
  Constant6 : Constant  Value=0  OutDataTypeStr=fixdt(0,1,0)  SampleTime=-1
  Delay : Delay  DelayLength=1  InitialCondition=0
  Delay1 : Delay  DelayLength=1  InitialCondition=0
  Delay2 : Delay  DelayLength=1  InitialCondition=0
  Extract Bits : simulink/Logic and Bit Operations/Extract Bits  bitsToExtract=Range starting with most significant bit  numBits=2  bitIdxRange=[6 7]  outScalingMode=Treat bit field as an integer
  Relational Operator1 : RelationalOperator  OutDataTypeStr=boolean  RndMeth=Simplest
  Subtract1 : Sum  Inputs=+-  OutDataTypeStr=Inherit: Inherit via back propagation
  Switch2 : Switch  Criteria=u2 > Threshold
  Switch4 : Switch  Criteria=u2 > Threshold
  shiftO : Outport
  RO : Outport  Port=2
  QO : Outport  Port=3
  wires:
  Delay2/1 -> QO/1
  Delay1/1 -> RO/1
  Delay/1 -> shiftO/1
  shiftI/1 -> Extract Bits/1, Delay/1
  Bit Concat1/1 -> Delay2/1
  Extract Bits/1 -> Subtract1/1, Switch2/3, Relational Operator1/1
  Subtract1/1 -> Switch2/1
  Relational Operator1/1 -> Switch2/2, Switch4/2
  Constant3/1 -> Switch4/3
  Constant6/1 -> Bit Concat1/1
  Constant2/1 -> Switch4/1
  Constant1/1 -> Relational Operator1/2, Subtract1/2
  Switch4/1 -> Bit Concat1/2
  Switch2/1 -> Delay1/1

== system CustArch_v22/cust_architecture/process_and_retrieve/spike_detection/LocalMaximaAdaptiveThreshold/RMS_computation/sqrt/sqrt_uint32/1_32bit/2_8bit/Subsystem1 ==
  shiftI : Inport
  RI : Inport  Port=2
  QI : Inport  Port=3
  Bit Concat5 : hdlsllib/Logic and Bit Operations/Bit Concat  numInputs=2
  Bit Concat8 : hdlsllib/Logic and Bit Operations/Bit Concat  numInputs=3
  Bit Concat9 : hdlsllib/Logic and Bit Operations/Bit Concat  numInputs=2
  Constant13 : Constant  Value=0  OutDataTypeStr=fixdt(0,1,0)  SampleTime=-1
  Constant14 : Constant  Value=0  OutDataTypeStr=fixdt(0,1,0)  SampleTime=-1
  Constant15 : Constant  OutDataTypeStr=fixdt(0,2,0)  SampleTime=-1
  Constant16 : Constant  OutDataTypeStr=fixdt(0,1,0)  SampleTime=-1
  Delay : Delay  DelayLength=1  InitialCondition=0
  Delay5 : Delay  DelayLength=1  InitialCondition=0
  Delay6 : Delay  DelayLength=1  InitialCondition=0
  Extract Bits3 : simulink/Logic and Bit Operations/Extract Bits  bitsToExtract=Range starting with most significant bit  numBits=2  bitIdxRange=[6 7]  outScalingMode=Treat bit field as an integer
  Relational Operator4 : RelationalOperator  OutDataTypeStr=boolean  RndMeth=Simplest
  Shift Arithmetic7 : ArithShift  BitShiftNumber=2  BitShiftDirection=Left
  Subtract4 : Sum  Inputs=+-  OutDataTypeStr=Inherit: Inherit via back propagation
  Switch8 : Switch  Criteria=u2 > Threshold
  Switch9 : Switch  Criteria=u2 > Threshold
  shiftO : Outport
  RO : Outport  Port=2
  QO : Outport  Port=3
  wires:
  Delay6/1 -> QO/1
  Delay5/1 -> RO/1
  Delay/1 -> shiftO/1
  Shift Arithmetic7/1 -> Extract Bits3/1, Delay/1
  Bit Concat5/1 -> Relational Operator4/1, Subtract4/1, Switch8/3
  Subtract4/1 -> Switch8/1
  Relational Operator4/1 -> Switch8/2, Switch9/2
  Bit Concat8/1 -> Delay6/1
  Switch8/1 -> Delay5/1
  RI/1 -> Bit Concat5/1
  Constant16/1 -> Switch9/1
  Constant13/1 -> Switch9/3
  Extract Bits3/1 -> Bit Concat5/2
  Bit Concat9/1 -> Relational Operator4/2, Subtract4/2
  Constant14/1 -> Bit Concat8/1
  shiftI/1 -> Shift Arithmetic7/1
  Constant15/1 -> Bit Concat9/2
  QI/1 -> Bit Concat9/1, Bit Concat8/2
  Switch9/1 -> Bit Concat8/3

== system CustArch_v22/cust_architecture/process_and_retrieve/spike_detection/LocalMaximaAdaptiveThreshold/RMS_computation/sqrt/sqrt_uint32/1_32bit/2_8bit/Subsystem2 ==
  shiftI : Inport
  RI : Inport  Port=2
  QI : Inport  Port=3
  Bit Concat5 : hdlsllib/Logic and Bit Operations/Bit Concat  numInputs=2
  Bit Concat8 : hdlsllib/Logic and Bit Operations/Bit Concat  numInputs=3
  Bit Concat9 : hdlsllib/Logic and Bit Operations/Bit Concat  numInputs=2
  Constant13 : Constant  Value=0  OutDataTypeStr=fixdt(0,1,0)  SampleTime=-1
  Constant14 : Constant  Value=0  OutDataTypeStr=fixdt(0,1,0)  SampleTime=-1
  Constant15 : Constant  OutDataTypeStr=fixdt(0,2,0)  SampleTime=-1
  Constant16 : Constant  OutDataTypeStr=fixdt(0,1,0)  SampleTime=-1
  Delay : Delay  DelayLength=1  InitialCondition=0
  Delay5 : Delay  DelayLength=1  InitialCondition=0
  Delay6 : Delay  DelayLength=1  InitialCondition=0
  Extract Bits3 : simulink/Logic and Bit Operations/Extract Bits  bitsToExtract=Range starting with most significant bit  numBits=2  bitIdxRange=[6 7]  outScalingMode=Treat bit field as an integer
  Relational Operator4 : RelationalOperator  OutDataTypeStr=boolean  RndMeth=Simplest
  Shift Arithmetic7 : ArithShift  BitShiftNumber=2  BitShiftDirection=Left
  Subtract4 : Sum  Inputs=+-  OutDataTypeStr=Inherit: Inherit via back propagation
  Switch8 : Switch  Criteria=u2 > Threshold
  Switch9 : Switch  Criteria=u2 > Threshold
  shiftO : Outport
  RO : Outport  Port=2
  QO : Outport  Port=3
  wires:
  Delay6/1 -> QO/1
  Delay5/1 -> RO/1
  Delay/1 -> shiftO/1
  Shift Arithmetic7/1 -> Extract Bits3/1, Delay/1
  Bit Concat5/1 -> Relational Operator4/1, Subtract4/1, Switch8/3
  Subtract4/1 -> Switch8/1
  Relational Operator4/1 -> Switch8/2, Switch9/2
  Bit Concat8/1 -> Delay6/1
  Switch8/1 -> Delay5/1
  RI/1 -> Bit Concat5/1
  Constant16/1 -> Switch9/1
  Constant13/1 -> Switch9/3
  Extract Bits3/1 -> Bit Concat5/2
  Bit Concat9/1 -> Relational Operator4/2, Subtract4/2
  Constant14/1 -> Bit Concat8/1
  shiftI/1 -> Shift Arithmetic7/1
  Constant15/1 -> Bit Concat9/2
  QI/1 -> Bit Concat9/1, Bit Concat8/2
  Switch9/1 -> Bit Concat8/3

== system CustArch_v22/cust_architecture/process_and_retrieve/spike_detection/LocalMaximaAdaptiveThreshold/RMS_computation/sqrt/sqrt_uint32/1_32bit/2_8bit/Subsystem3 ==
  shiftI : Inport
  RI : Inport  Port=2
  QI : Inport  Port=3
  Bit Concat5 : hdlsllib/Logic and Bit Operations/Bit Concat  numInputs=2
  Bit Concat8 : hdlsllib/Logic and Bit Operations/Bit Concat  numInputs=3
  Bit Concat9 : hdlsllib/Logic and Bit Operations/Bit Concat  numInputs=2
  Constant13 : Constant  Value=0  OutDataTypeStr=fixdt(0,1,0)  SampleTime=-1
  Constant14 : Constant  Value=0  OutDataTypeStr=fixdt(0,1,0)  SampleTime=-1
  Constant15 : Constant  OutDataTypeStr=fixdt(0,2,0)  SampleTime=-1
  Constant16 : Constant  OutDataTypeStr=fixdt(0,1,0)  SampleTime=-1
  Delay : Delay  DelayLength=1  InitialCondition=0
  Delay5 : Delay  DelayLength=1  InitialCondition=0
  Delay6 : Delay  DelayLength=1  InitialCondition=0
  Extract Bits3 : simulink/Logic and Bit Operations/Extract Bits  bitsToExtract=Range starting with most significant bit  numBits=2  bitIdxRange=[6 7]  outScalingMode=Treat bit field as an integer
  Relational Operator4 : RelationalOperator  OutDataTypeStr=boolean  RndMeth=Simplest
  Shift Arithmetic7 : ArithShift  BitShiftNumber=2  BitShiftDirection=Left
  Subtract4 : Sum  Inputs=+-  OutDataTypeStr=Inherit: Inherit via back propagation
  Switch8 : Switch  Criteria=u2 > Threshold
  Switch9 : Switch  Criteria=u2 > Threshold
  shiftO : Outport
  RO : Outport  Port=2
  QO : Outport  Port=3
  wires:
  Delay6/1 -> QO/1
  Delay5/1 -> RO/1
  Delay/1 -> shiftO/1
  Shift Arithmetic7/1 -> Extract Bits3/1, Delay/1
  Bit Concat5/1 -> Relational Operator4/1, Subtract4/1, Switch8/3
  Subtract4/1 -> Switch8/1
  Relational Operator4/1 -> Switch8/2, Switch9/2
  Bit Concat8/1 -> Delay6/1
  Switch8/1 -> Delay5/1
  RI/1 -> Bit Concat5/1
  Constant16/1 -> Switch9/1
  Constant13/1 -> Switch9/3
  Extract Bits3/1 -> Bit Concat5/2
  Bit Concat9/1 -> Relational Operator4/2, Subtract4/2
  Constant14/1 -> Bit Concat8/1
  shiftI/1 -> Shift Arithmetic7/1
  Constant15/1 -> Bit Concat9/2
  QI/1 -> Bit Concat9/1, Bit Concat8/2
  Switch9/1 -> Bit Concat8/3
